simulink model "RedCrane_kinematic_model"  (R2024a)
settings: Solver=FixedStepAuto  StartTime=0.0  StopTime=20  FixedStep=Ts  MaxStep=0.005  RelTol=1e-3
values from neighbouring files (symbols this model uses):
  M = [1, 0, 0, (L5 + L4 - L1) ... (first row only)    [enviroment_setup.m]
  SList = [ws_mat ... (first row only)    [enviroment_setup.m]
  telescope0 = 0    [enviroment_setup.m]
  thetaList0 = [0, 0,-pi/8, 0, 0]'    [enviroment_setup.m]
  Ts = 0.001    [enviroment_setup.m]
undefined symbols (not defined in the file or in its folder): dp_k_angle_to_stroke, dp_m_angle_to_stroke, p_k_angle_to_stroke, p_k_stroke_to_angle, p_m_angle_to_stroke, p_m_stroke_to_angle, X, Y, Z
libraries: sm_lib x82, nesl_utility x19, fl_lib x16
(part 3 of 3)

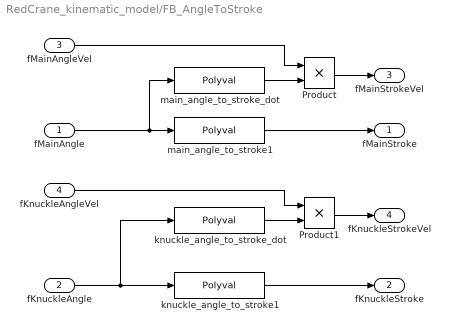
== system RedCrane_kinematic_model/FB_AngleToStroke ==
  fMainAngle : Inport
  fKnuckleAngle : Inport  Port=2
  fMainAngleVel : Inport  Port=3
  fKnuckleAngleVel : Inport  Port=4
  Product : Product
  Product1 : Product
  knuckle_angle_to_stroke1 : Polyval  Coefs=p_k_angle_to_stroke
  knuckle_angle_to_stroke_dot : Polyval  Coefs=dp_k_angle_to_stroke
  main_angle_to_stroke1 : Polyval  Coefs=p_m_angle_to_stroke
  main_angle_to_stroke_dot : Polyval  Coefs=dp_m_angle_to_stroke
  fMainStroke : Outport
  fKnuckleStroke : Outport  Port=2
  fMainStrokeVel : Outport  Port=3
  fKnuckleStrokeVel : Outport  Port=4
  wires:
  fMainAngle/1 -> main_angle_to_stroke_dot/1, main_angle_to_stroke1/1
  knuckle_angle_to_stroke_dot/1 -> Product1/2
  fKnuckleAngleVel/1 -> Product1/1
  fKnuckleAngle/1 -> knuckle_angle_to_stroke_dot/1, knuckle_angle_to_stroke1/1
  knuckle_angle_to_stroke1/1 -> fKnuckleStroke/1
  main_angle_to_stroke_dot/1 -> Product/2
  main_angle_to_stroke1/1 -> fMainStroke/1
  Product1/1 -> fKnuckleStrokeVel/1
  Product/1 -> fMainStrokeVel/1
  fMainAngleVel/1 -> Product/1

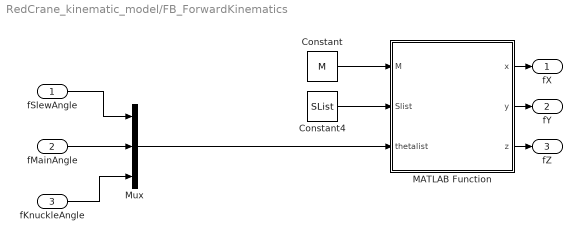
== system RedCrane_kinematic_model/FB_ForwardKinematics ==
  fSlewAngle : Inport
  fMainAngle : Inport  Port=2
  fKnuckleAngle : Inport  Port=3
  Constant : Constant  Value=M
  Constant4 : Constant  Value=SList
  MATLAB Function : MATLAB Function  TreatAsAtomicUnit=on
  Mux : Mux  Inputs=3
  fX : Outport
  fY : Outport  Port=2
  fZ : Outport  Port=3
  wires:
  MATLAB Function/1(x) -> fX/1
  Constant/1 -> MATLAB Function/1(M)
  Constant4/1 -> MATLAB Function/2(Slist)
  Mux/1 -> MATLAB Function/3(thetalist)
  MATLAB Function/3(z) -> fZ/1
  MATLAB Function/2(y) -> fY/1
  fSlewAngle/1 -> Mux/1
  fMainAngle/1 -> Mux/2
  fKnuckleAngle/1 -> Mux/3

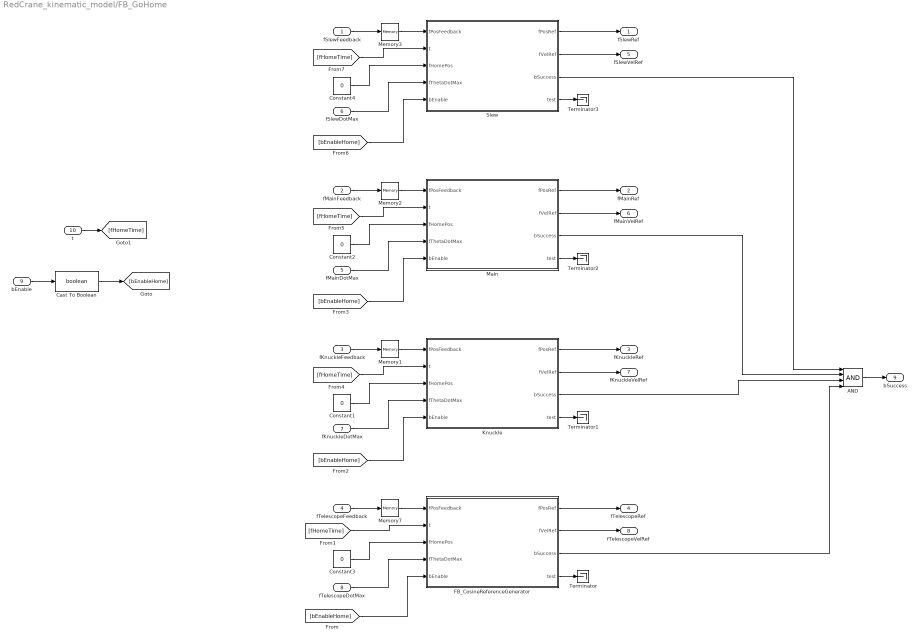
== system RedCrane_kinematic_model/FB_GoHome ==
  fSlewFeedback : Inport
  fMainFeedback : Inport  Port=2
  fKnuckleFeedback : Inport  Port=3
  fTelescopeFeedback : Inport  Port=4
  fMainDotMax : Inport  Port=5
  fSlewDotMax : Inport  Port=6
  fKnuckleDotMax : Inport  Port=7
  fTelescopeDotMax : Inport  Port=8
  bEnable : Inport  Port=9
  t : Inport  Port=10
  AND : Logic  Inputs=4  IconShape=distinctive  AllPortsSameDT=off  OutDataTypeStr=boolean
  Cast To Boolean : DataTypeConversion  OutDataTypeStr=boolean  SaturateOnIntegerOverflow=off  RndMeth=Floor
  Constant{1..4} (4 alike) : Constant  Value=0
  FB_CosineReferenceGenerator : MATLAB Function  TreatAsAtomicUnit=on
  Knuckle : MATLAB Function  TreatAsAtomicUnit=on
  Main : MATLAB Function  TreatAsAtomicUnit=on
  Memory1 : Memory  InitialCondition=thetaList0(3)
  Memory2 : Memory  InitialCondition=thetaList0(2)
  Memory3 : Memory  InitialCondition=thetaList0(1)
  Memory7 : Memory  InitialCondition=telescope0
  Slew : MATLAB Function  TreatAsAtomicUnit=on
  Terminator{,1..3} (4 alike) : Terminator
  fSlewRef : Outport
  fMainRef : Outport  Port=2
  fKnuckleRef : Outport  Port=3
  fTelescopeRef : Outport  Port=4
  fSlewVelRef : Outport  Port=5
  fMainVelRef : Outport  Port=6
  fKnuckleVelRef : Outport  Port=7
  fTelescopeVelRef : Outport  Port=8
  bSuccess : Outport  Port=9
  wires:
  FB_CosineReferenceGenerator/1(fPosRef) -> fTelescopeRef/1
  FB_CosineReferenceGenerator/3(bSuccess) -> AND/4
  [fHomeTime] -> FB_CosineReferenceGenerator/2(t)
  fTelescopeDotMax/1 -> FB_CosineReferenceGenerator/4(fThetaDotMax)
  [bEnableHome] -> FB_CosineReferenceGenerator/5(bEnable)
  fTelescopeFeedback/1 -> Memory7/1
  Constant3/1 -> FB_CosineReferenceGenerator/3(fHomePos)
  Memory7/1 -> FB_CosineReferenceGenerator/1(fPosFeedback)
  FB_CosineReferenceGenerator/2(fVelRef) -> fTelescopeVelRef/1
  FB_CosineReferenceGenerator/4(test) -> Terminator/1
  Constant1/1 -> Knuckle/3(fHomePos)
  Knuckle/3(bSuccess) -> AND/3
  Knuckle/2(fVelRef) -> fKnuckleVelRef/1
  Memory1/1 -> Knuckle/1(fPosFeedback)
  Knuckle/4(test) -> Terminator1/1
  Knuckle/1(fPosRef) -> fKnuckleRef/1
  [bEnableHome] -> Knuckle/5(bEnable)
  fKnuckleDotMax/1 -> Knuckle/4(fThetaDotMax)
  [fHomeTime] -> Knuckle/2(t)
  fKnuckleFeedback/1 -> Memory1/1
  AND/1 -> bSuccess/1
  bEnable/1 -> Cast To Boolean/1
  t/1 -> [fHomeTime]
  Cast To Boolean/1 -> [bEnableHome]
  Main/3(bSuccess) -> AND/2
  fMainDotMax/1 -> Main/4(fThetaDotMax)
  Main/4(test) -> Terminator2/1
  fMainFeedback/1 -> Memory2/1
  Memory2/1 -> Main/1(fPosFeedback)
  Main/2(fVelRef) -> fMainVelRef/1
  [bEnableHome] -> Main/5(bEnable)
  Constant2/1 -> Main/3(fHomePos)
  Main/1(fPosRef) -> fMainRef/1
  [fHomeTime] -> Main/2(t)
  [bEnableHome] -> Slew/5(bEnable)
  Slew/2(fVelRef) -> fSlewVelRef/1
  Memory3/1 -> Slew/1(fPosFeedback)
  Slew/3(bSuccess) -> AND/1
  Slew/4(test) -> Terminator3/1
  [fHomeTime] -> Slew/2(t)
  Slew/1(fPosRef) -> fSlewRef/1
  fSlewFeedback/1 -> Memory3/1
  Constant4/1 -> Slew/3(fHomePos)
  fSlewDotMax/1 -> Slew/4(fThetaDotMax)

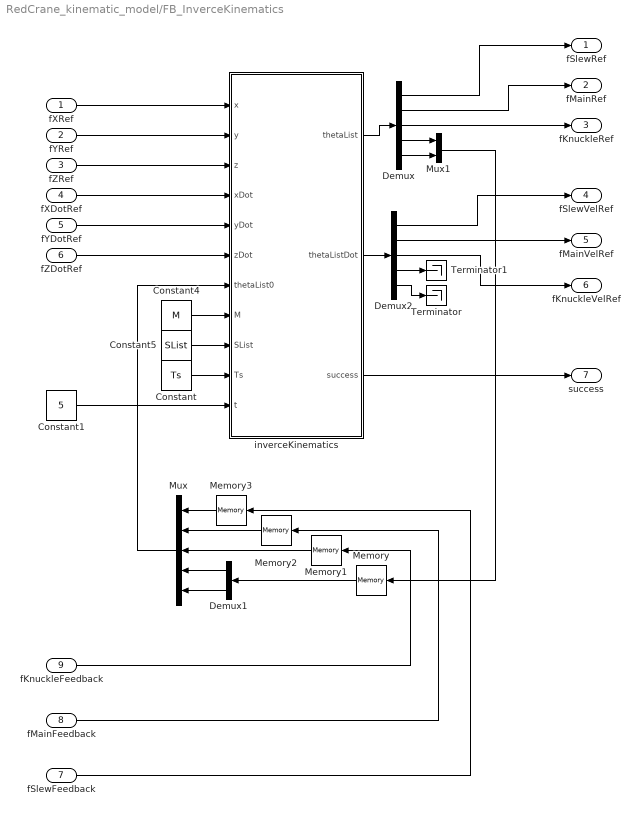
== system RedCrane_kinematic_model/FB_InverceKinematics ==
  fXRef : Inport
  fYRef : Inport  Port=2
  fZRef : Inport  Port=3
  fXDotRef : Inport  Port=4
  fYDotRef : Inport  Port=5
  fZDotRef : Inport  Port=6
  fSlewFeedback : Inport  Port=7
  fMainFeedback : Inport  Port=8
  fKnuckleFeedback : Inport  Port=9
  Constant : Constant  Value=Ts
  Constant1 : Constant  Value=5
  Constant4 : Constant  Value=M
  Constant5 : Constant  Value=SList
  Demux : Demux  Outputs=5
  Demux1 : Demux  Outputs=2
  Demux2 : Demux  Outputs=5
  Memory : Memory  InitialCondition=[thetaList0(4), thetaList0(5)]'
  Memory1 : Memory  InitialCondition=thetaList0(3)
  Memory2 : Memory  InitialCondition=thetaList0(2)
  Memory3 : Memory  InitialCondition=thetaList0(1)
  Mux : Mux  Inputs=5
  Mux1 : Mux  Inputs=2
  Terminator : Terminator
  Terminator1 : Terminator
  inverceKinematics : MATLAB Function  TreatAsAtomicUnit=on
  fSlewRef : Outport
  fMainRef : Outport  Port=2
  fKnuckleRef : Outport  Port=3
  fSlewVelRef : Outport  Port=4
  fMainVelRef : Outport  Port=5
  fKnuckleVelRef : Outport  Port=6
  success : Outport  Port=7
  wires:
  Memory1/1 -> Mux/3
  Demux/5 -> Mux1/2
  Constant4/1 -> inverceKinematics/8(M)
  Memory3/1 -> Mux/1
  Demux2/5 -> Terminator/1
  fSlewFeedback/1 -> Memory3/1
  Demux1/2 -> Mux/5
  Memory2/1 -> Mux/2
  Constant5/1 -> inverceKinematics/9(SList)
  Demux2/1 -> fSlewVelRef/1
  fXDotRef/1 -> inverceKinematics/4(xDot)
  inverceKinematics/1(thetaList) -> Demux/1
  Constant1/1 -> inverceKinematics/11(t)
  Demux/1 -> fSlewRef/1
  fXRef/1 -> inverceKinematics/1(x)
  Constant/1 -> inverceKinematics/10(Ts)
  Demux1/1 -> Mux/4
  Mux/1 -> inverceKinematics/7(thetaList0)
  Mux1/1 -> Memory/1
  fZRef/1 -> inverceKinematics/3(z)
  Memory/1 -> Demux1/1
  inverceKinematics/2(thetaListDot) -> Demux2/1
  Demux/4 -> Mux1/1
  Demux2/4 -> Terminator1/1
  fMainFeedback/1 -> Memory2/1
  fYRef/1 -> inverceKinematics/2(y)
  fKnuckleFeedback/1 -> Memory1/1
  Demux/3 -> fKnuckleRef/1
  fYDotRef/1 -> inverceKinematics/5(yDot)
  fZDotRef/1 -> inverceKinematics/6(zDot)
  Demux2/3 -> fKnuckleVelRef/1
  Demux/2 -> fMainRef/1
  Demux2/2 -> fMainVelRef/1
  inverceKinematics/3(success) -> success/1

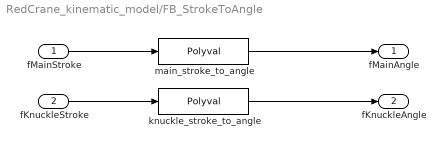
== system RedCrane_kinematic_model/FB_StrokeToAngle ==
  fMainStroke : Inport
  fKnuckleStroke : Inport  Port=2
  knuckle_stroke_to_angle : Polyval  Coefs=p_k_stroke_to_angle
  main_stroke_to_angle : Polyval  Coefs=p_m_stroke_to_angle
  fMainAngle : Outport
  fKnuckleAngle : Outport  Port=2
  wires:
  fKnuckleStroke/1 -> knuckle_stroke_to_angle/1
  fMainStroke/1 -> main_stroke_to_angle/1
  main_stroke_to_angle/1 -> fMainAngle/1
  knuckle_stroke_to_angle/1 -> fKnuckleAngle/1

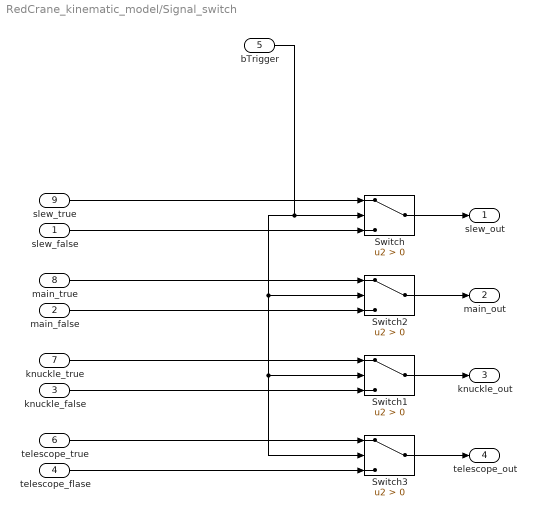
== system RedCrane_kinematic_model/Signal_switch ==
  slew_false : Inport
  main_false : Inport  Port=2
  knuckle_false : Inport  Port=3
  telescope_flase : Inport  Port=4
  bTrigger : Inport  Port=5
  telescope_true : Inport  Port=6
  knuckle_true : Inport  Port=7
  main_true : Inport  Port=8
  slew_true : Inport  Port=9
  Switch{,1..3} (4 alike) : Switch  Criteria=u2 > Threshold  SaturateOnIntegerOverflow=off  InputSameDT=off
  slew_out : Outport
  main_out : Outport  Port=2
  knuckle_out : Outport  Port=3
  telescope_out : Outport  Port=4
  wires:
  Switch1/1 -> knuckle_out/1
  bTrigger/1 -> Switch2/2, Switch1/2, Switch3/2, Switch/2
  telescope_true/1 -> Switch3/1
  slew_false/1 -> Switch/3
  Switch2/1 -> main_out/1
  slew_true/1 -> Switch/1
  knuckle_true/1 -> Switch1/1
  Switch3/1 -> telescope_out/1
  main_false/1 -> Switch2/3
  Switch/1 -> slew_out/1
  telescope_flase/1 -> Switch3/3
  knuckle_false/1 -> Switch1/3
  main_true/1 -> Switch2/1

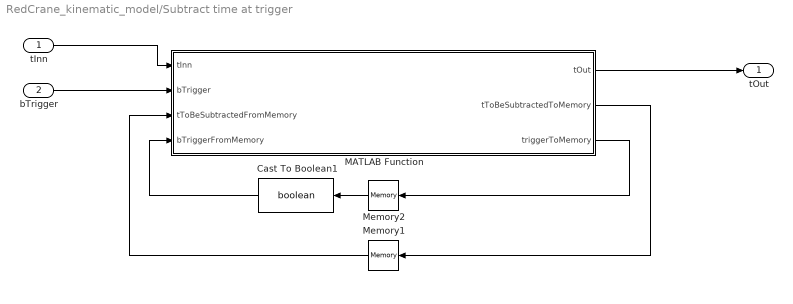
== system RedCrane_kinematic_model/Subtract time at trigger ==
  tInn : Inport
  bTrigger : Inport  Port=2
  Cast To Boolean1 : DataTypeConversion  OutDataTypeStr=boolean  SaturateOnIntegerOverflow=off  RndMeth=Floor
  MATLAB Function : MATLAB Function  TreatAsAtomicUnit=on
  Memory1 : Memory  InitialCondition=0.0
  Memory2 : Memory  InitialCondition=false
  tOut : Outport
  wires:
  MATLAB Function/2(tToBeSubtractedToMemory) -> Memory1/1
  Memory1/1 -> MATLAB Function/3(tToBeSubtractedFromMemory)
  MATLAB Function/1(tOut) -> tOut/1
  tInn/1 -> MATLAB Function/1(tInn)
  Memory2/1 -> Cast To Boolean1/1
  MATLAB Function/3(triggerToMemory) -> Memory2/1
  Cast To Boolean1/1 -> MATLAB Function/4(bTriggerFromMemory)
  bTrigger/1 -> MATLAB Function/2(bTrigger)

== matlab function RedCrane_kinematic_model/Subtract time at trigger/MATLAB Function ==
  data: tInn input; tOut output; bTrigger input; tToBeSubtractedFromMemory input; tToBeSubtractedToMemory output; bTriggerFromMemory input; triggerToMemory output
function [tOut, tToBeSubtractedToMemory, triggerToMemory] = subtractTimeFromRiseOfTrigger(tInn, bTrigger, tToBeSubtractedFromMemory, bTriggerFromMemory)

tToBeSubtractedToMemory = 0;
tOut = 0.0;

flag = false;
if(bTrigger & ~bTriggerFromMemory)
    tToBeSubtractedToMemory = tInn;
    flag = true;
else
    tToBeSubtractedToMemory = tToBeSubtractedFromMemory;
end



if(bTrigger)
    tOut = tInn - tToBeSubtractedFromMemory;
else
    tOut = 0.0;
end


% For smooting time when triggerd
if(flag)
    tOut = 0.0;
end

triggerToMemory = bTrigger;

== matlab function RedCrane_kinematic_model/FB_ForwardKinematics/MATLAB Function ==
  data: x output; M input; y output; Slist input; thetalist input; z output
function [x, y, z] = forvardKinematics(M, Slist, thetalist)
T = zeros(4, 4);
T = FKinSpace(M, Slist, thetalist);

x = T(1, 4);
y = T(2, 4);
z = T(3, 4);

== matlab function RedCrane_kinematic_model/FB_GoHome/Knuckle ==
  settings: updateMethod=DISCRETE
  data: fPosRef output; fVelRef output; fPosFeedback input; t input; fHomePos input; bSuccess output; fThetaDotMax input; bEnable input; test output
function [fPosRef, fVelRef, bSuccess, test] = goHomeKnuckle(fPosFeedback, ...
    t,...
    fHomePos,...
    fThetaDotMax, ...
    bEnable)

bSuccess = false;
fPosRef = 0.0;
fVelRef = 0.0;
test = false;




[fPosRef, fVelRef, bSuccess, test] = cosinePositionGenerator(fPosFeedback, fHomePos, fThetaDotMax, t, bEnable);



end

== matlab function RedCrane_kinematic_model/FB_InverceKinematics/inverceKinematics ==
  data: x input; thetaList output size=[5, 1]; y input; z input; xDot input; yDot input; zDot input; thetaList0 input; M input; SList input; Ts input; thetaListDot output size=[5, 1]; success output size=1; t input
function [thetaList, thetaListDot, success] = inverceKinematics( ...
    x, y, z, xDot, yDot, zDot, thetaList0, M, SList, Ts, t)

if(t <= Ts*1.1)
    thetaList0 = [0, 0, 0, 0, 0]';
end

% Explicitly pre-assign outputs
thetaList    = zeros(5,1);
thetaListDot = zeros(5,1);
success      = false;    % or 0 if you prefer numeric


T = [1 0 0 x;
    0 1 0 y;
    0 0 1 z;
    0 0 0 1];


[thetaOut, successOut] = IKinSpace(SList, M, T, thetaList0, 0.00001, 0.0000001);

% Assign them to the pre-allocated outputs
thetaList    = thetaOut;
success      = successOut;


Js = JacobianSpace(SList,thetaList);
Js_pinv = pinv(Js);
xyzDot = [0;
         0;
         0;
         xDot;
         yDot;
         zDot
         ];

thetaListDot = Js_pinv*xyzDot;

end

== matlab function RedCrane_kinematic_model/FB_GoHome/Main ==
  settings: updateMethod=DISCRETE
  data: fPosRef output; fVelRef output; fPosFeedback input; t input; fHomePos input; bSuccess output; fThetaDotMax input; bEnable input; test output
function [fPosRef, fVelRef, bSuccess, test] = goHomeMain(fPosFeedback, ...
    t,...
    fHomePos,...
    fThetaDotMax, ...
    bEnable)

bSuccess = false;
fPosRef = 0.0;
fVelRef = 0.0;
test = false;




[fPosRef, fVelRef, bSuccess, test] = cosinePositionGenerator(fPosFeedback, fHomePos, fThetaDotMax, t, bEnable);



end

== matlab function RedCrane_kinematic_model/FB_GoHome/Slew ==
  settings: updateMethod=DISCRETE
  data: fPosRef output; fVelRef output; fPosFeedback input; t input; fHomePos input; bSuccess output; fThetaDotMax input; bEnable input; test output
function [fPosRef, fVelRef, bSuccess, test] = goHomeSlew(fPosFeedback, ...
    t,...
    fHomePos,...
    fThetaDotMax, ...
    bEnable)

bSuccess = false;
fPosRef = 0.0;
fVelRef = 0.0;
test = false;




[fPosRef, fVelRef, bSuccess, test] = cosinePositionGenerator(fPosFeedback, fHomePos, fThetaDotMax, t, bEnable);



end

== matlab function RedCrane_kinematic_model/FB_GoHome/FB_CosineReferenceGenerator ==
  settings: updateMethod=DISCRETE
  data: fPosRef output; fVelRef output; fPosFeedback input; t input; fHomePos input; bSuccess output; fThetaDotMax input; bEnable input; test output
function [fPosRef, fVelRef, bSuccess, test] = goHomeTelescope(fPosFeedback, ...
    t,...
    fHomePos,...
    fThetaDotMax, ...
    bEnable)

bSuccess = false;
fPosRef = 0.0;
fVelRef = 0.0;
test = false;


[fPosRef, fVelRef, bSuccess, test] = cosinePositionGenerator(fPosFeedback, fHomePos, fThetaDotMax, t, bEnable);



end

== matlab function RedCrane_kinematic_model/MATLAB Function3 ==
  data: x output; y output; z output; t_current input; x_t output; y_t output; z_t output
function [x, y, z, x_t, y_t, z_t] = CubicPlanner(t_current)

% Position (xyz) and time vectors
px = [4.55, 0, 2];
py = [0.4, 3, 1];
pz = [1.6,  1.6,  2];
t =  [0,  5,  8];

if(t_current >= t(end))
    t_current = t(end);
end


%palpha = [0 0 0 0 pi/4 0 0];

pt = [px; py; pz]';

v = 0.005;

vx = [0 v 0];
vy = [0 v 0];
vz = [0 v 0];

if(t_current < t(2))
    idx = 1;
elseif(t_current < t(3))
    idx = 2;
else
    idx = 2;
end


t0 = t(idx);

x0 = pt(idx,  1);
x1 = pt(idx+1,1);
y0 = pt(idx,  2);
y1 = pt(idx+1,2);
z0 = pt(idx,  3);
z1 = pt(idx+1,3);

v0_x = vx(idx);
v1_x = vx(idx+1);

v0_y = vy(idx);
v1_y = vy(idx+1);

v0_z = vz(idx);
v1_z = vz(idx+1);

%alpha0 = palpha(idx);
%alpha1 = palpha(idx+1);

t1 = t(idx+1);
if(t_current < t(length(px)))
[x, x_t] = CubicRT(t0, t1, t_current, x0, x1, v0_x, v1_x);
[y, y_t] = CubicRT(t0, t1, t_current, y0, y1, v0_y, v1_y);
[z, z_t] = CubicRT(t0, t1, t_current, z0, z1, v0_z, v1_z);
%[alpha, alpha_t] = QuinticRT(t0, t1, t_current, alpha0, alpha1, 0, 0.001);
else
x = px(length(px));
y = py(length(py));
z = pz(length(pz));
x_t = 0;
y_t = 0;
z_t = 0;
%alpha_t = 0;
end
